simulink model "sixWheelModel"  (R2020b)
settings: Solver=VariableStepAuto  StartTime=0.0  StopTime=4  RelTol=1e-3
values from neighbouring files (symbols this model uses):
  mass = 1    [editvars.m]    (also in rovervars.mat)
  massRover = 50    [editvars.m]    (also in rovervars.mat)
  radius = 0.1    [editvars.m]    (also in rovervars.mat)
  stepTime = 2    [editvars.m]    (also in rovervars.mat)
  torqueF = 0.05    [editvars.m]    (also in rovervars.mat)
libraries: fl_lib x21, sdl_lib x13, nesl_utility x4
settings Model: Creator=lemck  LastModifiedBy=lemck

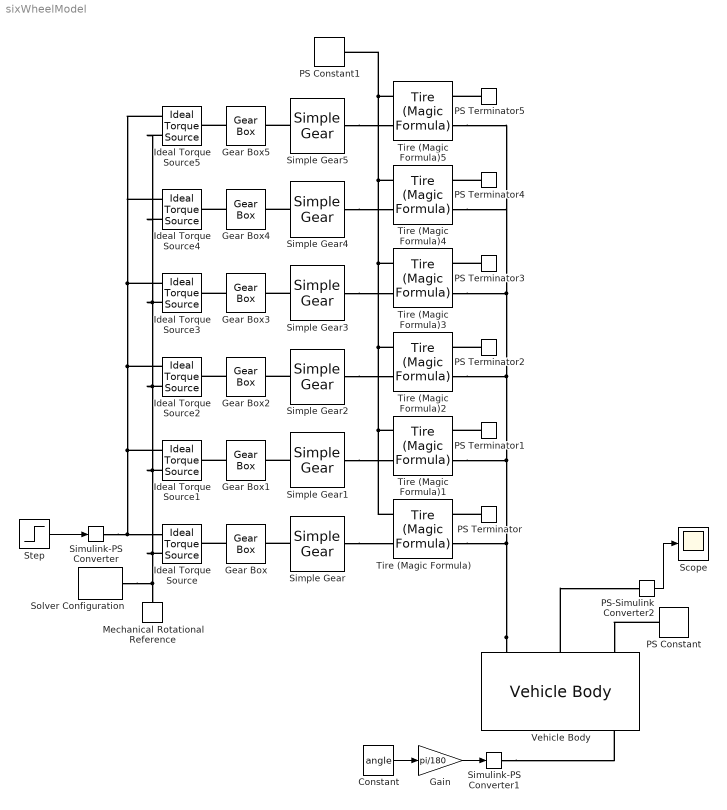
== system sixWheelModel ==
  Constant : Constant  Value=angle
  Gain : Gain  Gain=pi/180
  Gear Box{,1..5} (6 alike) : fl_lib/Mechanical/Mechanisms/Gear Box  ratio=100  t_in_specify=off  t_in_priority=None  t_in=0 N*m  t_in_nominal_specify=off  t_in_nominal_unit=N*m  t_in_nominal_value=1  t_out_specify=off  t_out_priority=None  t_out=0 N*m  t_out_nominal_specify=off  t_out_nominal_unit=N*m  t_out_nominal_value=1
  Ideal Torque Source{,1..5} (6 alike) : fl_lib/Mechanical/Mechanical Sources/Ideal Torque Source
  Mechanical Rotational Reference : fl_lib/Mechanical/Rotational Elements/Mechanical Rotational Reference
  PS Constant : fl_lib/Physical Signals/Sources/PS Constant  constant=windSpeed m/s
  PS Constant1 : fl_lib/Physical Signals/Sources/PS Constant  constant=massRover*9.81/6 N
  PS Terminator{,1..5} (6 alike) : fl_lib/Physical Signals/Sinks/PS Terminator
  PS-Simulink Converter2 : nesl_utility/PS-Simulink Converter  PhysicalDomain=network_engine_domain  SubClassName=ps_output  LeftPortType=input  RightPortType=output  PseudoPeriodic=off  Frequencies=[]  Unit=inherit  AffineConversion=off
  Scope : Scope
  Simple Gear{,1..5} (6 alike) : sdl_lib/Gears/Simple Gear  ratio=1  rotation_direction=sdl.enum.shaftOutputDirection.same  friction_model=sdl.enum.gear_efficiencies_load.constant  mu_visc=[0, 0] N*m/(rad/s)  T_noload=0.1 N*m  T_nom=5 N*m  efficiency_nom=0.8  efficiency=0.8  temperature_TLU=[280, 300, 320] K  load_TLU=[1, 5, 10] N*m  efficiency_TLU=[.95, .9, .85]  efficiency_TLU2=[.85, .8, .75; .95, .9, .85; .85, .8, .7]  w_thr=0.01 rad/s  pwr_thr=0.001 W  thermal_mass=50 J/K  enable_faults=simscape.enum.onoff.off  efficiency_fault=0.05  external_fault=simscape.enum.onoff.off  temporal_fault=simscape.enum.onoff.off  fault_time=5 s  fault_angles=pi / 12 rad  report_fault=simscape.enum.assert.action.none  temperature_specify=off  temperature_priority=High  temperature=300 K  temperature_nominal_specify=off  temperature_nominal_unit=K  temperature_nominal_value=1
  Simulink-PS Converter : nesl_utility/Simulink-PS Converter  PhysicalDomain=network_engine_domain  SubClassName=ps_input  LeftPortType=input  RightPortType=output  PseudoPeriodic=off  Frequencies=[]  NoiseDistribution=none  NoiseParameters=[]  Unit=1  AffineConversion=off  FilteringAndDerivatives=provide  SimscapeFilterOrder=1  InputFilterTimeConstant=0.001  UdotUserProvided=0
  Simulink-PS Converter1 : nesl_utility/Simulink-PS Converter  PhysicalDomain=network_engine_domain  SubClassName=ps_input  LeftPortType=input  RightPortType=output  PseudoPeriodic=off  Frequencies=[]  NoiseDistribution=none  NoiseParameters=[]  Unit=1  AffineConversion=off  FilteringAndDerivatives=provide  SimscapeFilterOrder=1  InputFilterTimeConstant=0.001  UdotUserProvided=0
  Solver Configuration : nesl_utility/Solver Configuration  PhysicalDomain=network_engine_domain  SubClassName=solver  LeftPortType=input  RightPortType=generic  Tones=[]  Harmonics=[]  SimulateNoise=off  Profile=off  UseLocalSampling=off  EnableSwitchedLinearOptims=on  FrequencyDomain=off  UseCCode=off  RelTol=0.001  AbsTol=1e-06  MinStep=1e-09  ToWorkspace=off  RevertToSquareIcSolve=off  NumHomotopyIterations=100  PhasorMode=off  PhasorModeNumHarmonics=1  DoDC=off  ResidualTolerance=1e-09  UseLocalSolver=off  LocalSolverChoice=NE_BACKWARD_EULER_ADVANCER  LocalSolverSampleTime=0.001  DoFixedCost=off  MaxNonlinIter=3  MaxModeIter=2  ComputeImpulses=off  ImpulseIterations=2  LinearAlgebra=auto  EquationFormulation=NE_TIME_EF  DelaysMemoryBudget=1024  AutomaticFiltering=on  FilteringTimeConstant=0.001  PartitionStorageMethod=AS_NEEDED  PartitionMemoryBudget=1024  PartitionMethod=ROBUST
  Step : Step  Time=stepTime  After=torqueF  SampleTime=0
  Tire (Magic Formula){,1..5} (6 alike) : sdl_lib/Tires & Vehicles/Tire (Magic Formula)  parameterization=sdl.enum.magic_tire_model.constant  F_z1=3000 N  F_x1=3500 N  kappa1=10  B_m=12  C_m=2.3  D_m=0.82  E_m=1  fz0=4000 N  p_Cx=1.685  p_Dx=[1.21, -.037]  p_Ex=[.344, .095, -.02, 0]  p_Kx=[21.51, -.163, .245]  p_Hx=[-.002, .002]  p_Vx=[0, 0]  v_tr_thr=0.1 m/s  r_e=radius m  model_compliance=0  stiffness=1e6 N/m  damping=1000 N/(m/s)  model_inertia=1  inertia=mass*radius^2 kg*m^2  initial_velocity=0 rad/s  model_resistance=0  resistance_model=1  coeff=0.015  p_tire=250e3 Pa  alpha=-0.003  beta=0.97  coeff_a=84e-4  coeff_b=6.2e-4 s/m  coeff_c=1.6e-4 s^2/m^2  v_thr=0.001 m/s
  Vehicle Body : sdl_lib/Tires & Vehicles/Vehicle Body  mass=massRover kg  n_w=2  x_f=1.4 m  x_r=1.6 m  y_c=0.5 m  mass_var=simscape.enum.onoff.off  model_pitch=simscape.enum.onoff.off  inertia=4000 kg*m^2  suspension_model=sdl.enum.linearTLU.linear  k_f=1e4 N/m  b_f=1e4 N/(m/s)  k_r=1e4 N/m  b_r=1e4 N/(m/s)  k_f_TLU=[-2000, -1000, 0, 1000, 2000] N  x_f_TLU=[-.4, -.2, 0, .2, .4] m  b_f_TLU=[-200, -100, 0, 100, 200] N  v_f_TLU=[-4, -2, 0, 2, 4] m/s  k_r_TLU=[-2000, -1000, 0, 1000, 2000] N  x_r_TLU=[-.4, -.2, 0, .2, .4] m  b_r_TLU=[-200, -100, 0, 100, 200] N  v_r_TLU=[-4, -2, 0, 2, 4] m/s  interp_method=simscape.enum.interpolation.linear  extrap_method=simscape.enum.extrapolation.linear  model_hardstop=simscape.enum.onoff.off  upper_bound_f=.25 m  lower_bound_f=-.25 m  stop_k_f=1e6 N/m  stop_b_f=150 N/(m/s)  upper_bound_r=.25 m  lower_bound_r=-.25 m  stop_k_r=1e6 N/m  stop_b_r=150 N/(m/s)  initial_pitch=0 rad  initial_pitch_rate=0 rad/s  g=9.81 m/s^2  liftoff_warning=simscape.enum.onoff.off  area=area m^2  Cd=2.1  rho=1.18 kg/m^3  v_specify=off  v_priority=High  v=0 m/s  v_nominal_specify=off  v_nominal_unit=m/s  v_nominal_value=1
  wires:
  Step/1 -> Simulink-PS Converter/1
  Constant/1 -> Gain/1
  Gain/1 -> Simulink-PS Converter1/1
  PS-Simulink Converter2/1 -> Scope/1
  connections:
  Vehicle Body/LConn1 -- Tire (Magic Formula)5/RConn2 -- Tire (Magic Formula)4/RConn2 -- Tire (Magic Formula)3/RConn2 -- Tire (Magic Formula)2/RConn2 -- Tire (Magic Formula)1/RConn2 -- Tire (Magic Formula)/RConn2
  Ideal Torque Source/RConn2 -- Ideal Torque Source5/RConn2 -- Ideal Torque Source4/RConn2 -- Ideal Torque Source3/RConn2 -- Ideal Torque Source2/RConn2 -- Ideal Torque Source1/RConn2 -- Solver Configuration/RConn1 -- Mechanical Rotational Reference/LConn1
  Simulink-PS Converter/RConn1 -- Ideal Torque Source2/RConn1 -- Ideal Torque Source5/RConn1 -- Ideal Torque Source4/RConn1 -- Ideal Torque Source3/RConn1 -- Ideal Torque Source1/RConn1 -- Ideal Torque Source/RConn1
  Vehicle Body/LConn2 -- PS-Simulink Converter2/LConn1
  PS Constant/RConn1 -- Vehicle Body/LConn3
  Simulink-PS Converter1/RConn1 -- Vehicle Body/RConn3
  Tire (Magic Formula)/LConn1 -- Tire (Magic Formula)1/LConn1 -- Tire (Magic Formula)4/LConn1 -- Tire (Magic Formula)5/LConn1 -- PS Constant1/RConn1 -- Tire (Magic Formula)3/LConn1 -- Tire (Magic Formula)2/LConn1
  PS Terminator/LConn1 -- Tire (Magic Formula)/RConn1
  Gear Box/LConn1 -- Ideal Torque Source/LConn1
  Simple Gear/LConn1 -- Gear Box/RConn1
  Simple Gear/RConn1 -- Tire (Magic Formula)/LConn2
  PS Terminator1/LConn1 -- Tire (Magic Formula)1/RConn1
  Gear Box1/LConn1 -- Ideal Torque Source1/LConn1
  Simple Gear1/RConn1 -- Tire (Magic Formula)1/LConn2
  Simple Gear1/LConn1 -- Gear Box1/RConn1
  PS Terminator2/LConn1 -- Tire (Magic Formula)2/RConn1
  Gear Box2/LConn1 -- Ideal Torque Source2/LConn1
  Simple Gear2/RConn1 -- Tire (Magic Formula)2/LConn2
  Simple Gear2/LConn1 -- Gear Box2/RConn1
  PS Terminator3/LConn1 -- Tire (Magic Formula)3/RConn1
  Gear Box3/LConn1 -- Ideal Torque Source3/LConn1
  Simple Gear3/RConn1 -- Tire (Magic Formula)3/LConn2
  Simple Gear3/LConn1 -- Gear Box3/RConn1
  PS Terminator4/LConn1 -- Tire (Magic Formula)4/RConn1
  Gear Box4/LConn1 -- Ideal Torque Source4/LConn1
  Simple Gear4/RConn1 -- Tire (Magic Formula)4/LConn2
  Simple Gear4/LConn1 -- Gear Box4/RConn1
  PS Terminator5/LConn1 -- Tire (Magic Formula)5/RConn1
  Gear Box5/LConn1 -- Ideal Torque Source5/LConn1
  Simple Gear5/RConn1 -- Tire (Magic Formula)5/LConn2
  Simple Gear5/LConn1 -- Gear Box5/RConn1
